simulink model "robot_action"  (R2014b)
settings: Solver=ode45  StartTime=0.0  StopTime=10  FixedStep=1e-4  RelTol=1e-3
values from neighbouring files (symbols this model uses):
  robot_floor_friction_coeff = 0.6    [robot_init.m]
  robot_floor_position_gain = -1e5    (= -100000)    [robot_init.m]
  robot_floor_speed_gain = -1e3    (= -1000)    [robot_init.m]
  robot_gravity = [0 0 -9.80665]    [robot_init.m]
undefined symbols (not defined in the file or in its folder): CM730_acc_center, CM730_acc_gain, CM730_gyro_center, CM730_gyro_gain, CM730_sample_time, FSR_max, FSR_no_load, FSR_sample_time, FSR_scale, MX28_inertia, MX28_Te, X, Y, Z
libraries: sm_lib x158, fl_lib x128, nesl_utility x77
(part 5 of 6)

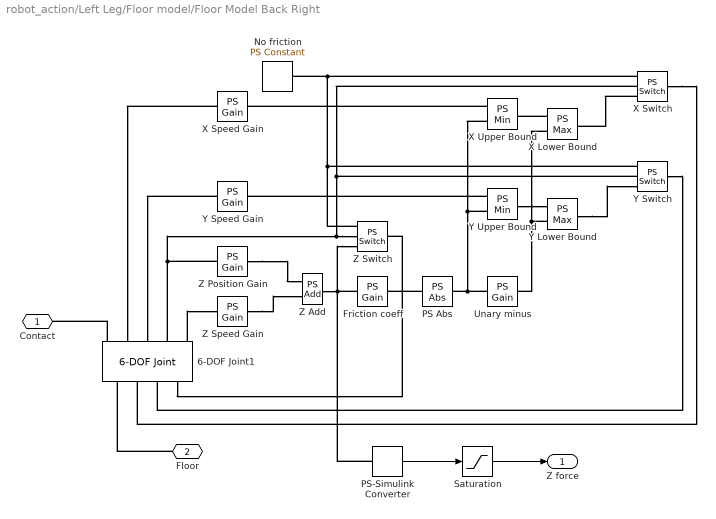
== system robot_action/Left Leg/Floor model/Floor Model Back Right ==
  6-DOF Joint1 : sm_lib/Joints/6-DOF Joint  SenseConstraintForce=off  SenseConstraintForceX=off  SenseConstraintForceY=off  SenseConstraintForceZ=off  SenseConstraintTorque=off  SenseConstraintTorqueX=off  SenseConstraintTorqueY=off  SenseConstraintTorqueZ=off  SenseTotalForce=off  SenseTotalForceX=off  SenseTotalForceY=off  SenseTotalForceZ=off  SenseTotalTorque=off  SenseTotalTorqueX=off  SenseTotalTorqueY=off  SenseTotalTorqueZ=off  CompositeWrenchDir=FollowerOnBase  CompositeWrenchFrame=BaseFrame  PxEquilibriumPosition=0  PxEquilibriumPositionUnits=m  PxSpringStiffness=0  PxSpringStiffnessUnits=N/m  PxDampingCoefficient=0  PxDampingCoefficientUnits=N/(m/s)  PxTorqueActuationMode=InputTorque  PxMotionActuationMode=ComputedMotion  PxSensePosition=off  PxSenseVelocity=on  PxSenseAcceleration=off  PxSenseTorqueForce=off  PxPositionTargetValue=0  PxPositionTargetValueUnits=m  PxPositionTargetSpecify=off  PxPositionTargetPriority=High  PxVelocityTargetValue=0  PxVelocityTargetValueUnits=m/s  PxVelocityTargetSpecify=off  PxVelocityTargetPriority=High  PyEquilibriumPosition=0  PyEquilibriumPositionUnits=m  PySpringStiffness=0  PySpringStiffnessUnits=N/m  PyDampingCoefficient=0  PyDampingCoefficientUnits=N/(m/s)  PyTorqueActuationMode=InputTorque  PyMotionActuationMode=ComputedMotion  PySensePosition=off  PySenseVelocity=on  PySenseAcceleration=off  PySenseTorqueForce=off  PyPositionTargetValue=0  PyPositionTargetValueUnits=m  PyPositionTargetSpecify=off  PyPositionTargetPriority=High  PyVelocityTargetValue=0  PyVelocityTargetValueUnits=m/s  PyVelocityTargetSpecify=off  PyVelocityTargetPriority=High  PzEquilibriumPosition=0  PzEquilibriumPositionUnits=m  PzSpringStiffness=0  PzSpringStiffnessUnits=N/m  PzDampingCoefficient=0  PzDampingCoefficientUnits=N/(m/s)  PzTorqueActuationMode=InputTorque  PzMotionActuationMode=ComputedMotion  PzSensePosition=on  PzSenseVelocity=on  PzSenseAcceleration=off  PzSenseTorqueForce=off  PzPositionTargetValue=0  PzPositionTargetValueUnits=m  PzPositionTargetSpecify=off  PzPositionTargetPriority=High  PzVelocityTargetValue=0  PzVelocityTargetValueUnits=m/s  PzVelocityTargetSpecify=off  PzVelocityTargetPriority=High  SphDefPosRotationMethod=None  SphDefPosRotationAngleUnits=deg  SphDefPosRotationStandardAxis=+Z  SphDefPosRotationAngle=0.0  SphDefPosRotationArbitraryAxis=[0 0 1]  SphDefPosFollAlignAxisA=+X  SphDefPosBaseAlignAxisA=+Y  SphDefPosFollAlignAxisB=+Y  SphDefPosBaseAlignAxisB=+Z  SphDefPosRotationMatrix=[1 0 0; 0 1 0; 0 0 1]  SphEqPosRotationMethod=None  SphEqPosRotationAngleUnits=deg  SphEqPosRotationStandardAxis=+Z  SphEqPosRotationAngle=0.0  SphEqPosRotationArbitraryAxis=[0 0 1]  SphEqPosFollAlignAxisA=+X  SphEqPosBaseAlignAxisA=+Y  SphEqPosFollAlignAxisB=+Y  SphEqPosBaseAlignAxisB=+Z  SphEqPosRotationMatrix=[1 0 0; 0 1 0; 0 0 1]  SphSpringStiffness=0  SphSpringStiffnessUnits=N*m/deg  SphDampingCoefficient=0  SphDampingCoefficientUnits=N*m/(deg/s)  SphActuateTorqueX=off  SphActuateTorqueY=off  SphActuateTorqueZ=off  SphActuateTorque=off  SphTorqueActuationMode=NoTorque  SphMotionActuationMode=ComputedMotion  SphActuationFrame=BaseFrame  SphSensePosition=off  SphSenseVelocityX=off  SphSenseVelocityY=off  SphSenseVelocityZ=off  SphSenseVelocity=off  SphSenseAccelerationX=off  SphSenseAccelerationY=off  SphSenseAccelerationZ=off  SphSenseAcceleration=off  SphSenseTorqueX=off  SphSenseTorqueY=off  SphSenseTorqueZ=off  SphSenseTorqueForce=off  SphSensingFrame=BaseFrame  SphPositionTargetRotationMethod=None  SphPositionTargetRotationAngleUnits=deg  SphPositionTargetRotationStandardAxis=+Z  SphPositionTargetRotationAngle=0.0  SphPositionTargetRotationArbitraryAxis=[0 0 1]  SphPositionTargetFollAlignAxisA=+X  SphPositionTargetBaseAlignAxisA=+Y  SphPositionTargetFollAlignAxisB=+Y  SphPositionTargetBaseAlignAxisB=+Z  SphPositionTargetRotationMatrix=[1 0 0; 0 1 0; 0 0 1]  SphPositionTargetSpecify=off  SphPositionTargetPriority=High  SphVelocityTargetValue=[0 0 0]  SphVelocityTargetValueUnits=deg/s  SphVelocityTargetSpecify=off  SphVelocityTargetPriority=High  SphVelocityTargetInFollowerFrame=on  BlockFunction=simmechanics.library.joints.sixdof_joint
  Friction coeff : fl_lib/Physical Signals/Functions/PS Gain  gain=robot_floor_friction_coeff
  No friction : fl_lib/Physical Signals/Sources/PS Constant  constant=0
  PS Abs : fl_lib/Physical Signals/Nonlinear Operators/PS Abs
  PS-Simulink Converter : nesl_utility/PS-Simulink Converter  PhysicalDomain=network_engine_domain  SubClassName=ps_output  LeftPortType=input  RightPortType=output  PseudoPeriodic=off  Frequencies=[]  Unit=N  AffineConversion=off
  Saturation : Saturate  UpperLimit=+inf  LowerLimit=0
  Unary minus : fl_lib/Physical Signals/Functions/PS Gain  gain=-1
  X Lower Bound : fl_lib/Physical Signals/Nonlinear Operators/PS Max
  X Speed Gain : fl_lib/Physical Signals/Functions/PS Gain  gain=robot_floor_speed_gain
  X Switch : fl_lib/Physical Signals/Nonlinear Operators/PS Switch  Threshold=0
  X Upper Bound : fl_lib/Physical Signals/Nonlinear Operators/PS Min
  Y Lower Bound : fl_lib/Physical Signals/Nonlinear Operators/PS Max
  Y Speed Gain : fl_lib/Physical Signals/Functions/PS Gain  gain=robot_floor_speed_gain
  Y Switch : fl_lib/Physical Signals/Nonlinear Operators/PS Switch  Threshold=0
  Y Upper Bound : fl_lib/Physical Signals/Nonlinear Operators/PS Min
  Z Add : fl_lib/Physical Signals/Functions/PS Add
  Z Position Gain : fl_lib/Physical Signals/Functions/PS Gain  gain=robot_floor_position_gain
  Z Speed Gain : fl_lib/Physical Signals/Functions/PS Gain  gain=robot_floor_speed_gain
  Z Switch : fl_lib/Physical Signals/Nonlinear Operators/PS Switch  Threshold=0
  Contact : PMIOPort  Port=1  Side=Left
  Floor : PMIOPort  Port=2  Side=Right
  Z force : Outport
  wires:
  PS-Simulink Converter/1 -> Saturation/1
  Saturation/1 -> Z force/1
  connections:
  Floor/RConn1 -- 6-DOF Joint1/LConn1
  6-DOF Joint1/RConn1 -- Contact/RConn1
  No friction/RConn1 -- Y Switch/LConn1 -- Z Switch/LConn1 -- X Switch/LConn1
  Z Position Gain/RConn1 -- Z Add/LConn1
  Z Switch/LConn3 -- Z Add/RConn1 -- Friction coeff/LConn1 -- PS-Simulink Converter/LConn1
  Z Speed Gain/RConn1 -- Z Add/LConn2
  6-DOF Joint1/RConn5 -- Z Speed Gain/LConn1
  6-DOF Joint1/LConn4 -- Z Switch/RConn1
  Z Switch/LConn2 -- Z Position Gain/LConn1 -- 6-DOF Joint1/RConn4 -- X Switch/LConn2 -- Y Switch/LConn2
  Y Switch/RConn1 -- 6-DOF Joint1/LConn3
  Y Speed Gain/LConn1 -- 6-DOF Joint1/RConn3
  PS Abs/LConn1 -- Friction coeff/RConn1
  PS Abs/RConn1 -- Unary minus/LConn1 -- X Upper Bound/LConn2 -- Y Upper Bound/LConn2
  Y Upper Bound/RConn1 -- Y Lower Bound/LConn1
  Y Lower Bound/LConn2 -- Unary minus/RConn1 -- X Lower Bound/LConn2
  Y Lower Bound/RConn1 -- Y Switch/LConn3
  Y Upper Bound/LConn1 -- Y Speed Gain/RConn1
  X Speed Gain/LConn1 -- 6-DOF Joint1/RConn2
  X Upper Bound/LConn1 -- X Speed Gain/RConn1
  X Lower Bound/LConn1 -- X Upper Bound/RConn1
  X Switch/LConn3 -- X Lower Bound/RConn1
  X Switch/RConn1 -- 6-DOF Joint1/LConn2

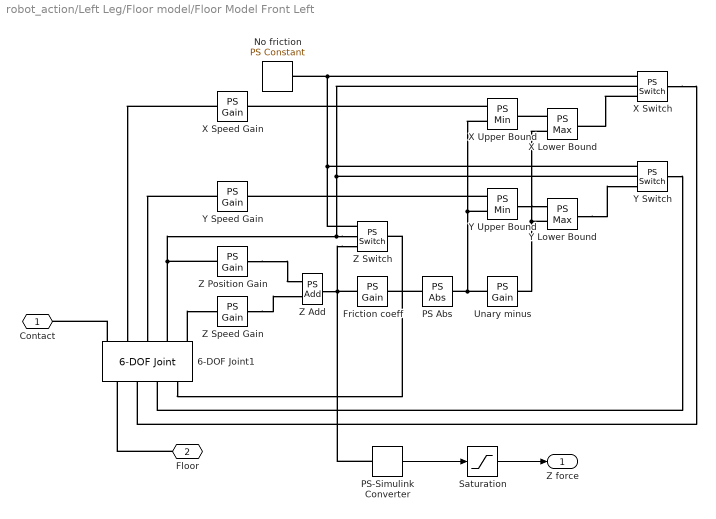
== system robot_action/Left Leg/Floor model/Floor Model Front Left ==
  6-DOF Joint1 : sm_lib/Joints/6-DOF Joint  SenseConstraintForce=off  SenseConstraintForceX=off  SenseConstraintForceY=off  SenseConstraintForceZ=off  SenseConstraintTorque=off  SenseConstraintTorqueX=off  SenseConstraintTorqueY=off  SenseConstraintTorqueZ=off  SenseTotalForce=off  SenseTotalForceX=off  SenseTotalForceY=off  SenseTotalForceZ=off  SenseTotalTorque=off  SenseTotalTorqueX=off  SenseTotalTorqueY=off  SenseTotalTorqueZ=off  CompositeWrenchDir=FollowerOnBase  CompositeWrenchFrame=BaseFrame  PxEquilibriumPosition=0  PxEquilibriumPositionUnits=m  PxSpringStiffness=0  PxSpringStiffnessUnits=N/m  PxDampingCoefficient=0  PxDampingCoefficientUnits=N/(m/s)  PxTorqueActuationMode=InputTorque  PxMotionActuationMode=ComputedMotion  PxSensePosition=off  PxSenseVelocity=on  PxSenseAcceleration=off  PxSenseTorqueForce=off  PxPositionTargetValue=0  PxPositionTargetValueUnits=m  PxPositionTargetSpecify=off  PxPositionTargetPriority=High  PxVelocityTargetValue=0  PxVelocityTargetValueUnits=m/s  PxVelocityTargetSpecify=off  PxVelocityTargetPriority=High  PyEquilibriumPosition=0  PyEquilibriumPositionUnits=m  PySpringStiffness=0  PySpringStiffnessUnits=N/m  PyDampingCoefficient=0  PyDampingCoefficientUnits=N/(m/s)  PyTorqueActuationMode=InputTorque  PyMotionActuationMode=ComputedMotion  PySensePosition=off  PySenseVelocity=on  PySenseAcceleration=off  PySenseTorqueForce=off  PyPositionTargetValue=0  PyPositionTargetValueUnits=m  PyPositionTargetSpecify=off  PyPositionTargetPriority=High  PyVelocityTargetValue=0  PyVelocityTargetValueUnits=m/s  PyVelocityTargetSpecify=off  PyVelocityTargetPriority=High  PzEquilibriumPosition=0  PzEquilibriumPositionUnits=m  PzSpringStiffness=0  PzSpringStiffnessUnits=N/m  PzDampingCoefficient=0  PzDampingCoefficientUnits=N/(m/s)  PzTorqueActuationMode=InputTorque  PzMotionActuationMode=ComputedMotion  PzSensePosition=on  PzSenseVelocity=on  PzSenseAcceleration=off  PzSenseTorqueForce=off  PzPositionTargetValue=0  PzPositionTargetValueUnits=m  PzPositionTargetSpecify=off  PzPositionTargetPriority=High  PzVelocityTargetValue=0  PzVelocityTargetValueUnits=m/s  PzVelocityTargetSpecify=off  PzVelocityTargetPriority=High  SphDefPosRotationMethod=None  SphDefPosRotationAngleUnits=deg  SphDefPosRotationStandardAxis=+Z  SphDefPosRotationAngle=0.0  SphDefPosRotationArbitraryAxis=[0 0 1]  SphDefPosFollAlignAxisA=+X  SphDefPosBaseAlignAxisA=+Y  SphDefPosFollAlignAxisB=+Y  SphDefPosBaseAlignAxisB=+Z  SphDefPosRotationMatrix=[1 0 0; 0 1 0; 0 0 1]  SphEqPosRotationMethod=None  SphEqPosRotationAngleUnits=deg  SphEqPosRotationStandardAxis=+Z  SphEqPosRotationAngle=0.0  SphEqPosRotationArbitraryAxis=[0 0 1]  SphEqPosFollAlignAxisA=+X  SphEqPosBaseAlignAxisA=+Y  SphEqPosFollAlignAxisB=+Y  SphEqPosBaseAlignAxisB=+Z  SphEqPosRotationMatrix=[1 0 0; 0 1 0; 0 0 1]  SphSpringStiffness=0  SphSpringStiffnessUnits=N*m/deg  SphDampingCoefficient=0  SphDampingCoefficientUnits=N*m/(deg/s)  SphActuateTorqueX=off  SphActuateTorqueY=off  SphActuateTorqueZ=off  SphActuateTorque=off  SphTorqueActuationMode=NoTorque  SphMotionActuationMode=ComputedMotion  SphActuationFrame=BaseFrame  SphSensePosition=off  SphSenseVelocityX=off  SphSenseVelocityY=off  SphSenseVelocityZ=off  SphSenseVelocity=off  SphSenseAccelerationX=off  SphSenseAccelerationY=off  SphSenseAccelerationZ=off  SphSenseAcceleration=off  SphSenseTorqueX=off  SphSenseTorqueY=off  SphSenseTorqueZ=off  SphSenseTorqueForce=off  SphSensingFrame=BaseFrame  SphPositionTargetRotationMethod=None  SphPositionTargetRotationAngleUnits=deg  SphPositionTargetRotationStandardAxis=+Z  SphPositionTargetRotationAngle=0.0  SphPositionTargetRotationArbitraryAxis=[0 0 1]  SphPositionTargetFollAlignAxisA=+X  SphPositionTargetBaseAlignAxisA=+Y  SphPositionTargetFollAlignAxisB=+Y  SphPositionTargetBaseAlignAxisB=+Z  SphPositionTargetRotationMatrix=[1 0 0; 0 1 0; 0 0 1]  SphPositionTargetSpecify=off  SphPositionTargetPriority=High  SphVelocityTargetValue=[0 0 0]  SphVelocityTargetValueUnits=deg/s  SphVelocityTargetSpecify=off  SphVelocityTargetPriority=High  SphVelocityTargetInFollowerFrame=on  BlockFunction=simmechanics.library.joints.sixdof_joint
  Friction coeff : fl_lib/Physical Signals/Functions/PS Gain  gain=robot_floor_friction_coeff
  No friction : fl_lib/Physical Signals/Sources/PS Constant  constant=0
  PS Abs : fl_lib/Physical Signals/Nonlinear Operators/PS Abs
  PS-Simulink Converter : nesl_utility/PS-Simulink Converter  PhysicalDomain=network_engine_domain  SubClassName=ps_output  LeftPortType=input  RightPortType=output  PseudoPeriodic=off  Frequencies=[]  Unit=N  AffineConversion=off
  Saturation : Saturate  UpperLimit=+inf  LowerLimit=0
  Unary minus : fl_lib/Physical Signals/Functions/PS Gain  gain=-1
  X Lower Bound : fl_lib/Physical Signals/Nonlinear Operators/PS Max
  X Speed Gain : fl_lib/Physical Signals/Functions/PS Gain  gain=robot_floor_speed_gain
  X Switch : fl_lib/Physical Signals/Nonlinear Operators/PS Switch  Threshold=0
  X Upper Bound : fl_lib/Physical Signals/Nonlinear Operators/PS Min
  Y Lower Bound : fl_lib/Physical Signals/Nonlinear Operators/PS Max
  Y Speed Gain : fl_lib/Physical Signals/Functions/PS Gain  gain=robot_floor_speed_gain
  Y Switch : fl_lib/Physical Signals/Nonlinear Operators/PS Switch  Threshold=0
  Y Upper Bound : fl_lib/Physical Signals/Nonlinear Operators/PS Min
  Z Add : fl_lib/Physical Signals/Functions/PS Add
  Z Position Gain : fl_lib/Physical Signals/Functions/PS Gain  gain=robot_floor_position_gain
  Z Speed Gain : fl_lib/Physical Signals/Functions/PS Gain  gain=robot_floor_speed_gain
  Z Switch : fl_lib/Physical Signals/Nonlinear Operators/PS Switch  Threshold=0
  Contact : PMIOPort  Port=1  Side=Left
  Floor : PMIOPort  Port=2  Side=Right
  Z force : Outport
  wires:
  PS-Simulink Converter/1 -> Saturation/1
  Saturation/1 -> Z force/1
  connections:
  Floor/RConn1 -- 6-DOF Joint1/LConn1
  6-DOF Joint1/RConn1 -- Contact/RConn1
  No friction/RConn1 -- Y Switch/LConn1 -- Z Switch/LConn1 -- X Switch/LConn1
  Z Position Gain/RConn1 -- Z Add/LConn1
  Z Switch/LConn3 -- PS-Simulink Converter/LConn1 -- Z Add/RConn1 -- Friction coeff/LConn1
  Z Speed Gain/RConn1 -- Z Add/LConn2
  6-DOF Joint1/RConn5 -- Z Speed Gain/LConn1
  6-DOF Joint1/LConn4 -- Z Switch/RConn1
  Z Switch/LConn2 -- Z Position Gain/LConn1 -- 6-DOF Joint1/RConn4 -- X Switch/LConn2 -- Y Switch/LConn2
  Y Switch/RConn1 -- 6-DOF Joint1/LConn3
  Y Speed Gain/LConn1 -- 6-DOF Joint1/RConn3
  PS Abs/LConn1 -- Friction coeff/RConn1
  PS Abs/RConn1 -- Unary minus/LConn1 -- X Upper Bound/LConn2 -- Y Upper Bound/LConn2
  Y Upper Bound/RConn1 -- Y Lower Bound/LConn1
  Y Lower Bound/LConn2 -- Unary minus/RConn1 -- X Lower Bound/LConn2
  Y Lower Bound/RConn1 -- Y Switch/LConn3
  Y Upper Bound/LConn1 -- Y Speed Gain/RConn1
  X Speed Gain/LConn1 -- 6-DOF Joint1/RConn2
  X Upper Bound/LConn1 -- X Speed Gain/RConn1
  X Lower Bound/LConn1 -- X Upper Bound/RConn1
  X Switch/LConn3 -- X Lower Bound/RConn1
  X Switch/RConn1 -- 6-DOF Joint1/LConn2

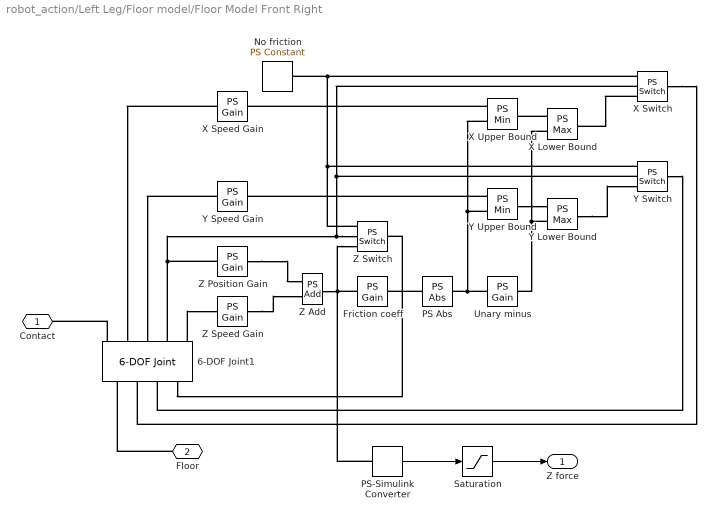
== system robot_action/Left Leg/Floor model/Floor Model Front Right ==
  6-DOF Joint1 : sm_lib/Joints/6-DOF Joint  SenseConstraintForce=off  SenseConstraintForceX=off  SenseConstraintForceY=off  SenseConstraintForceZ=off  SenseConstraintTorque=off  SenseConstraintTorqueX=off  SenseConstraintTorqueY=off  SenseConstraintTorqueZ=off  SenseTotalForce=off  SenseTotalForceX=off  SenseTotalForceY=off  SenseTotalForceZ=off  SenseTotalTorque=off  SenseTotalTorqueX=off  SenseTotalTorqueY=off  SenseTotalTorqueZ=off  CompositeWrenchDir=FollowerOnBase  CompositeWrenchFrame=BaseFrame  PxEquilibriumPosition=0  PxEquilibriumPositionUnits=m  PxSpringStiffness=0  PxSpringStiffnessUnits=N/m  PxDampingCoefficient=0  PxDampingCoefficientUnits=N/(m/s)  PxTorqueActuationMode=InputTorque  PxMotionActuationMode=ComputedMotion  PxSensePosition=off  PxSenseVelocity=on  PxSenseAcceleration=off  PxSenseTorqueForce=off  PxPositionTargetValue=0  PxPositionTargetValueUnits=m  PxPositionTargetSpecify=off  PxPositionTargetPriority=High  PxVelocityTargetValue=0  PxVelocityTargetValueUnits=m/s  PxVelocityTargetSpecify=off  PxVelocityTargetPriority=High  PyEquilibriumPosition=0  PyEquilibriumPositionUnits=m  PySpringStiffness=0  PySpringStiffnessUnits=N/m  PyDampingCoefficient=0  PyDampingCoefficientUnits=N/(m/s)  PyTorqueActuationMode=InputTorque  PyMotionActuationMode=ComputedMotion  PySensePosition=off  PySenseVelocity=on  PySenseAcceleration=off  PySenseTorqueForce=off  PyPositionTargetValue=0  PyPositionTargetValueUnits=m  PyPositionTargetSpecify=off  PyPositionTargetPriority=High  PyVelocityTargetValue=0  PyVelocityTargetValueUnits=m/s  PyVelocityTargetSpecify=off  PyVelocityTargetPriority=High  PzEquilibriumPosition=0  PzEquilibriumPositionUnits=m  PzSpringStiffness=0  PzSpringStiffnessUnits=N/m  PzDampingCoefficient=0  PzDampingCoefficientUnits=N/(m/s)  PzTorqueActuationMode=InputTorque  PzMotionActuationMode=ComputedMotion  PzSensePosition=on  PzSenseVelocity=on  PzSenseAcceleration=off  PzSenseTorqueForce=off  PzPositionTargetValue=0  PzPositionTargetValueUnits=m  PzPositionTargetSpecify=off  PzPositionTargetPriority=High  PzVelocityTargetValue=0  PzVelocityTargetValueUnits=m/s  PzVelocityTargetSpecify=off  PzVelocityTargetPriority=High  SphDefPosRotationMethod=None  SphDefPosRotationAngleUnits=deg  SphDefPosRotationStandardAxis=+Z  SphDefPosRotationAngle=0.0  SphDefPosRotationArbitraryAxis=[0 0 1]  SphDefPosFollAlignAxisA=+X  SphDefPosBaseAlignAxisA=+Y  SphDefPosFollAlignAxisB=+Y  SphDefPosBaseAlignAxisB=+Z  SphDefPosRotationMatrix=[1 0 0; 0 1 0; 0 0 1]  SphEqPosRotationMethod=None  SphEqPosRotationAngleUnits=deg  SphEqPosRotationStandardAxis=+Z  SphEqPosRotationAngle=0.0  SphEqPosRotationArbitraryAxis=[0 0 1]  SphEqPosFollAlignAxisA=+X  SphEqPosBaseAlignAxisA=+Y  SphEqPosFollAlignAxisB=+Y  SphEqPosBaseAlignAxisB=+Z  SphEqPosRotationMatrix=[1 0 0; 0 1 0; 0 0 1]  SphSpringStiffness=0  SphSpringStiffnessUnits=N*m/deg  SphDampingCoefficient=0  SphDampingCoefficientUnits=N*m/(deg/s)  SphActuateTorqueX=off  SphActuateTorqueY=off  SphActuateTorqueZ=off  SphActuateTorque=off  SphTorqueActuationMode=NoTorque  SphMotionActuationMode=ComputedMotion  SphActuationFrame=BaseFrame  SphSensePosition=off  SphSenseVelocityX=off  SphSenseVelocityY=off  SphSenseVelocityZ=off  SphSenseVelocity=off  SphSenseAccelerationX=off  SphSenseAccelerationY=off  SphSenseAccelerationZ=off  SphSenseAcceleration=off  SphSenseTorqueX=off  SphSenseTorqueY=off  SphSenseTorqueZ=off  SphSenseTorqueForce=off  SphSensingFrame=BaseFrame  SphPositionTargetRotationMethod=None  SphPositionTargetRotationAngleUnits=deg  SphPositionTargetRotationStandardAxis=+Z  SphPositionTargetRotationAngle=0.0  SphPositionTargetRotationArbitraryAxis=[0 0 1]  SphPositionTargetFollAlignAxisA=+X  SphPositionTargetBaseAlignAxisA=+Y  SphPositionTargetFollAlignAxisB=+Y  SphPositionTargetBaseAlignAxisB=+Z  SphPositionTargetRotationMatrix=[1 0 0; 0 1 0; 0 0 1]  SphPositionTargetSpecify=off  SphPositionTargetPriority=High  SphVelocityTargetValue=[0 0 0]  SphVelocityTargetValueUnits=deg/s  SphVelocityTargetSpecify=off  SphVelocityTargetPriority=High  SphVelocityTargetInFollowerFrame=on  BlockFunction=simmechanics.library.joints.sixdof_joint
  Friction coeff : fl_lib/Physical Signals/Functions/PS Gain  gain=robot_floor_friction_coeff
  No friction : fl_lib/Physical Signals/Sources/PS Constant  constant=0
  PS Abs : fl_lib/Physical Signals/Nonlinear Operators/PS Abs
  PS-Simulink Converter : nesl_utility/PS-Simulink Converter  PhysicalDomain=network_engine_domain  SubClassName=ps_output  LeftPortType=input  RightPortType=output  PseudoPeriodic=off  Frequencies=[]  Unit=N  AffineConversion=off
  Saturation : Saturate  UpperLimit=+inf  LowerLimit=0
  Unary minus : fl_lib/Physical Signals/Functions/PS Gain  gain=-1
  X Lower Bound : fl_lib/Physical Signals/Nonlinear Operators/PS Max
  X Speed Gain : fl_lib/Physical Signals/Functions/PS Gain  gain=robot_floor_speed_gain
  X Switch : fl_lib/Physical Signals/Nonlinear Operators/PS Switch  Threshold=0
  X Upper Bound : fl_lib/Physical Signals/Nonlinear Operators/PS Min
  Y Lower Bound : fl_lib/Physical Signals/Nonlinear Operators/PS Max
  Y Speed Gain : fl_lib/Physical Signals/Functions/PS Gain  gain=robot_floor_speed_gain
  Y Switch : fl_lib/Physical Signals/Nonlinear Operators/PS Switch  Threshold=0
  Y Upper Bound : fl_lib/Physical Signals/Nonlinear Operators/PS Min
  Z Add : fl_lib/Physical Signals/Functions/PS Add
  Z Position Gain : fl_lib/Physical Signals/Functions/PS Gain  gain=robot_floor_position_gain
  Z Speed Gain : fl_lib/Physical Signals/Functions/PS Gain  gain=robot_floor_speed_gain
  Z Switch : fl_lib/Physical Signals/Nonlinear Operators/PS Switch  Threshold=0
  Contact : PMIOPort  Port=1  Side=Left
  Floor : PMIOPort  Port=2  Side=Right
  Z force : Outport
  wires:
  PS-Simulink Converter/1 -> Saturation/1
  Saturation/1 -> Z force/1
  connections:
  Floor/RConn1 -- 6-DOF Joint1/LConn1
  6-DOF Joint1/RConn1 -- Contact/RConn1
  No friction/RConn1 -- Y Switch/LConn1 -- Z Switch/LConn1 -- X Switch/LConn1
  Z Position Gain/RConn1 -- Z Add/LConn1
  Z Switch/LConn3 -- Z Add/RConn1 -- Friction coeff/LConn1 -- PS-Simulink Converter/LConn1
  Z Speed Gain/RConn1 -- Z Add/LConn2
  6-DOF Joint1/RConn5 -- Z Speed Gain/LConn1
  6-DOF Joint1/LConn4 -- Z Switch/RConn1
  Z Switch/LConn2 -- Z Position Gain/LConn1 -- 6-DOF Joint1/RConn4 -- X Switch/LConn2 -- Y Switch/LConn2
  Y Switch/RConn1 -- 6-DOF Joint1/LConn3
  Y Speed Gain/LConn1 -- 6-DOF Joint1/RConn3
  PS Abs/LConn1 -- Friction coeff/RConn1
  PS Abs/RConn1 -- Unary minus/LConn1 -- X Upper Bound/LConn2 -- Y Upper Bound/LConn2
  Y Upper Bound/RConn1 -- Y Lower Bound/LConn1
  Y Lower Bound/LConn2 -- Unary minus/RConn1 -- X Lower Bound/LConn2
  Y Lower Bound/RConn1 -- Y Switch/LConn3
  Y Upper Bound/LConn1 -- Y Speed Gain/RConn1
  X Speed Gain/LConn1 -- 6-DOF Joint1/RConn2
  X Upper Bound/LConn1 -- X Speed Gain/RConn1
  X Lower Bound/LConn1 -- X Upper Bound/RConn1
  X Switch/LConn3 -- X Lower Bound/RConn1
  X Switch/RConn1 -- 6-DOF Joint1/LConn2

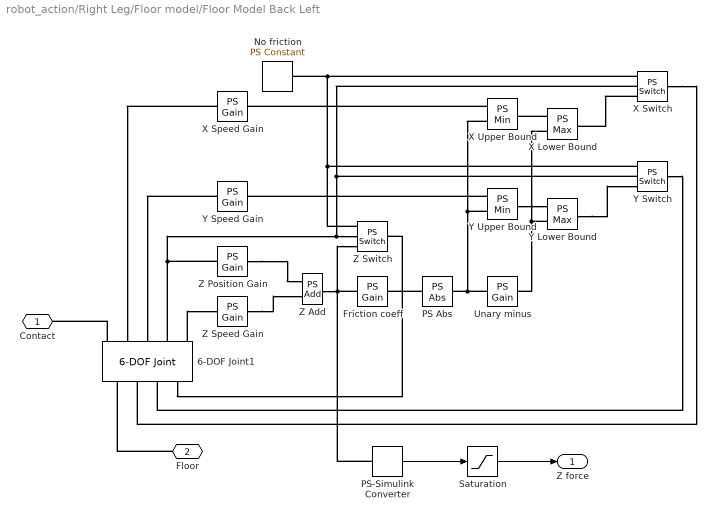
== system robot_action/Right Leg/Floor model/Floor Model Back Left ==
  6-DOF Joint1 : sm_lib/Joints/6-DOF Joint  SenseConstraintForce=off  SenseConstraintForceX=off  SenseConstraintForceY=off  SenseConstraintForceZ=off  SenseConstraintTorque=off  SenseConstraintTorqueX=off  SenseConstraintTorqueY=off  SenseConstraintTorqueZ=off  SenseTotalForce=off  SenseTotalForceX=off  SenseTotalForceY=off  SenseTotalForceZ=off  SenseTotalTorque=off  SenseTotalTorqueX=off  SenseTotalTorqueY=off  SenseTotalTorqueZ=off  CompositeWrenchDir=FollowerOnBase  CompositeWrenchFrame=BaseFrame  PxEquilibriumPosition=0  PxEquilibriumPositionUnits=m  PxSpringStiffness=0  PxSpringStiffnessUnits=N/m  PxDampingCoefficient=0  PxDampingCoefficientUnits=N/(m/s)  PxTorqueActuationMode=InputTorque  PxMotionActuationMode=ComputedMotion  PxSensePosition=off  PxSenseVelocity=on  PxSenseAcceleration=off  PxSenseTorqueForce=off  PxPositionTargetValue=0  PxPositionTargetValueUnits=m  PxPositionTargetSpecify=off  PxPositionTargetPriority=High  PxVelocityTargetValue=0  PxVelocityTargetValueUnits=m/s  PxVelocityTargetSpecify=off  PxVelocityTargetPriority=High  PyEquilibriumPosition=0  PyEquilibriumPositionUnits=m  PySpringStiffness=0  PySpringStiffnessUnits=N/m  PyDampingCoefficient=0  PyDampingCoefficientUnits=N/(m/s)  PyTorqueActuationMode=InputTorque  PyMotionActuationMode=ComputedMotion  PySensePosition=off  PySenseVelocity=on  PySenseAcceleration=off  PySenseTorqueForce=off  PyPositionTargetValue=0  PyPositionTargetValueUnits=m  PyPositionTargetSpecify=off  PyPositionTargetPriority=High  PyVelocityTargetValue=0  PyVelocityTargetValueUnits=m/s  PyVelocityTargetSpecify=off  PyVelocityTargetPriority=High  PzEquilibriumPosition=0  PzEquilibriumPositionUnits=m  PzSpringStiffness=0  PzSpringStiffnessUnits=N/m  PzDampingCoefficient=0  PzDampingCoefficientUnits=N/(m/s)  PzTorqueActuationMode=InputTorque  PzMotionActuationMode=ComputedMotion  PzSensePosition=on  PzSenseVelocity=on  PzSenseAcceleration=off  PzSenseTorqueForce=off  PzPositionTargetValue=0  PzPositionTargetValueUnits=m  PzPositionTargetSpecify=off  PzPositionTargetPriority=High  PzVelocityTargetValue=0  PzVelocityTargetValueUnits=m/s  PzVelocityTargetSpecify=off  PzVelocityTargetPriority=High  SphDefPosRotationMethod=None  SphDefPosRotationAngleUnits=deg  SphDefPosRotationStandardAxis=+Z  SphDefPosRotationAngle=0.0  SphDefPosRotationArbitraryAxis=[0 0 1]  SphDefPosFollAlignAxisA=+X  SphDefPosBaseAlignAxisA=+Y  SphDefPosFollAlignAxisB=+Y  SphDefPosBaseAlignAxisB=+Z  SphDefPosRotationMatrix=[1 0 0; 0 1 0; 0 0 1]  SphEqPosRotationMethod=None  SphEqPosRotationAngleUnits=deg  SphEqPosRotationStandardAxis=+Z  SphEqPosRotationAngle=0.0  SphEqPosRotationArbitraryAxis=[0 0 1]  SphEqPosFollAlignAxisA=+X  SphEqPosBaseAlignAxisA=+Y  SphEqPosFollAlignAxisB=+Y  SphEqPosBaseAlignAxisB=+Z  SphEqPosRotationMatrix=[1 0 0; 0 1 0; 0 0 1]  SphSpringStiffness=0  SphSpringStiffnessUnits=N*m/deg  SphDampingCoefficient=0  SphDampingCoefficientUnits=N*m/(deg/s)  SphActuateTorqueX=off  SphActuateTorqueY=off  SphActuateTorqueZ=off  SphActuateTorque=off  SphTorqueActuationMode=NoTorque  SphMotionActuationMode=ComputedMotion  SphActuationFrame=BaseFrame  SphSensePosition=off  SphSenseVelocityX=off  SphSenseVelocityY=off  SphSenseVelocityZ=off  SphSenseVelocity=off  SphSenseAccelerationX=off  SphSenseAccelerationY=off  SphSenseAccelerationZ=off  SphSenseAcceleration=off  SphSenseTorqueX=off  SphSenseTorqueY=off  SphSenseTorqueZ=off  SphSenseTorqueForce=off  SphSensingFrame=BaseFrame  SphPositionTargetRotationMethod=None  SphPositionTargetRotationAngleUnits=deg  SphPositionTargetRotationStandardAxis=+Z  SphPositionTargetRotationAngle=0.0  SphPositionTargetRotationArbitraryAxis=[0 0 1]  SphPositionTargetFollAlignAxisA=+X  SphPositionTargetBaseAlignAxisA=+Y  SphPositionTargetFollAlignAxisB=+Y  SphPositionTargetBaseAlignAxisB=+Z  SphPositionTargetRotationMatrix=[1 0 0; 0 1 0; 0 0 1]  SphPositionTargetSpecify=off  SphPositionTargetPriority=High  SphVelocityTargetValue=[0 0 0]  SphVelocityTargetValueUnits=deg/s  SphVelocityTargetSpecify=off  SphVelocityTargetPriority=High  SphVelocityTargetInFollowerFrame=on  BlockFunction=simmechanics.library.joints.sixdof_joint
  Friction coeff : fl_lib/Physical Signals/Functions/PS Gain  gain=robot_floor_friction_coeff
  No friction : fl_lib/Physical Signals/Sources/PS Constant  constant=0
  PS Abs : fl_lib/Physical Signals/Nonlinear Operators/PS Abs
  PS-Simulink Converter : nesl_utility/PS-Simulink Converter  PhysicalDomain=network_engine_domain  SubClassName=ps_output  LeftPortType=input  RightPortType=output  PseudoPeriodic=off  Frequencies=[]  Unit=N  AffineConversion=off
  Saturation : Saturate  UpperLimit=+inf  LowerLimit=0
  Unary minus : fl_lib/Physical Signals/Functions/PS Gain  gain=-1
  X Lower Bound : fl_lib/Physical Signals/Nonlinear Operators/PS Max
  X Speed Gain : fl_lib/Physical Signals/Functions/PS Gain  gain=robot_floor_speed_gain
  X Switch : fl_lib/Physical Signals/Nonlinear Operators/PS Switch  Threshold=0
  X Upper Bound : fl_lib/Physical Signals/Nonlinear Operators/PS Min
  Y Lower Bound : fl_lib/Physical Signals/Nonlinear Operators/PS Max
  Y Speed Gain : fl_lib/Physical Signals/Functions/PS Gain  gain=robot_floor_speed_gain
  Y Switch : fl_lib/Physical Signals/Nonlinear Operators/PS Switch  Threshold=0
  Y Upper Bound : fl_lib/Physical Signals/Nonlinear Operators/PS Min
  Z Add : fl_lib/Physical Signals/Functions/PS Add
  Z Position Gain : fl_lib/Physical Signals/Functions/PS Gain  gain=robot_floor_position_gain
  Z Speed Gain : fl_lib/Physical Signals/Functions/PS Gain  gain=robot_floor_speed_gain
  Z Switch : fl_lib/Physical Signals/Nonlinear Operators/PS Switch  Threshold=0
  Contact : PMIOPort  Port=1  Side=Left
  Floor : PMIOPort  Port=2  Side=Right
  Z force : Outport
  wires:
  PS-Simulink Converter/1 -> Saturation/1
  Saturation/1 -> Z force/1
  connections:
  Floor/RConn1 -- 6-DOF Joint1/LConn1
  6-DOF Joint1/RConn1 -- Contact/RConn1
  No friction/RConn1 -- Y Switch/LConn1 -- Z Switch/LConn1 -- X Switch/LConn1
  Z Position Gain/RConn1 -- Z Add/LConn1
  Z Switch/LConn3 -- Z Add/RConn1 -- Friction coeff/LConn1 -- PS-Simulink Converter/LConn1
  Z Speed Gain/RConn1 -- Z Add/LConn2
  6-DOF Joint1/RConn5 -- Z Speed Gain/LConn1
  6-DOF Joint1/LConn4 -- Z Switch/RConn1
  Z Switch/LConn2 -- Z Position Gain/LConn1 -- 6-DOF Joint1/RConn4 -- X Switch/LConn2 -- Y Switch/LConn2
  Y Switch/RConn1 -- 6-DOF Joint1/LConn3
  Y Speed Gain/LConn1 -- 6-DOF Joint1/RConn3
  PS Abs/LConn1 -- Friction coeff/RConn1
  PS Abs/RConn1 -- Unary minus/LConn1 -- X Upper Bound/LConn2 -- Y Upper Bound/LConn2
  Y Upper Bound/RConn1 -- Y Lower Bound/LConn1
  Y Lower Bound/LConn2 -- Unary minus/RConn1 -- X Lower Bound/LConn2
  Y Lower Bound/RConn1 -- Y Switch/LConn3
  Y Upper Bound/LConn1 -- Y Speed Gain/RConn1
  X Speed Gain/LConn1 -- 6-DOF Joint1/RConn2
  X Upper Bound/LConn1 -- X Speed Gain/RConn1
  X Lower Bound/LConn1 -- X Upper Bound/RConn1
  X Switch/LConn3 -- X Lower Bound/RConn1
  X Switch/RConn1 -- 6-DOF Joint1/LConn2

== system robot_action/Right Leg/Floor model/Floor Model Back Right ==
  6-DOF Joint1 : sm_lib/Joints/6-DOF Joint  SenseConstraintForce=off  SenseConstraintForceX=off  SenseConstraintForceY=off  SenseConstraintForceZ=off  SenseConstraintTorque=off  SenseConstraintTorqueX=off  SenseConstraintTorqueY=off  SenseConstraintTorqueZ=off  SenseTotalForce=off  SenseTotalForceX=off  SenseTotalForceY=off  SenseTotalForceZ=off  SenseTotalTorque=off  SenseTotalTorqueX=off  SenseTotalTorqueY=off  SenseTotalTorqueZ=off  CompositeWrenchDir=FollowerOnBase  CompositeWrenchFrame=BaseFrame  PxEquilibriumPosition=0  PxEquilibriumPositionUnits=m  PxSpringStiffness=0  PxSpringStiffnessUnits=N/m  PxDampingCoefficient=0  PxDampingCoefficientUnits=N/(m/s)  PxTorqueActuationMode=InputTorque  PxMotionActuationMode=ComputedMotion  PxSensePosition=off  PxSenseVelocity=on  PxSenseAcceleration=off  PxSenseTorqueForce=off  PxPositionTargetValue=0  PxPositionTargetValueUnits=m  PxPositionTargetSpecify=off  PxPositionTargetPriority=High  PxVelocityTargetValue=0  PxVelocityTargetValueUnits=m/s  PxVelocityTargetSpecify=off  PxVelocityTargetPriority=High  PyEquilibriumPosition=0  PyEquilibriumPositionUnits=m  PySpringStiffness=0  PySpringStiffnessUnits=N/m  PyDampingCoefficient=0  PyDampingCoefficientUnits=N/(m/s)  PyTorqueActuationMode=InputTorque  PyMotionActuationMode=ComputedMotion  PySensePosition=off  PySenseVelocity=on  PySenseAcceleration=off  PySenseTorqueForce=off  PyPositionTargetValue=0  PyPositionTargetValueUnits=m  PyPositionTargetSpecify=off  PyPositionTargetPriority=High  PyVelocityTargetValue=0  PyVelocityTargetValueUnits=m/s  PyVelocityTargetSpecify=off  PyVelocityTargetPriority=High  PzEquilibriumPosition=0  PzEquilibriumPositionUnits=m  PzSpringStiffness=0  PzSpringStiffnessUnits=N/m  PzDampingCoefficient=0  PzDampingCoefficientUnits=N/(m/s)  PzTorqueActuationMode=InputTorque  PzMotionActuationMode=ComputedMotion  PzSensePosition=on  PzSenseVelocity=on  PzSenseAcceleration=off  PzSenseTorqueForce=off  PzPositionTargetValue=0  PzPositionTargetValueUnits=m  PzPositionTargetSpecify=off  PzPositionTargetPriority=High  PzVelocityTargetValue=0  PzVelocityTargetValueUnits=m/s  PzVelocityTargetSpecify=off  PzVelocityTargetPriority=High  SphDefPosRotationMethod=None  SphDefPosRotationAngleUnits=deg  SphDefPosRotationStandardAxis=+Z  SphDefPosRotationAngle=0.0  SphDefPosRotationArbitraryAxis=[0 0 1]  SphDefPosFollAlignAxisA=+X  SphDefPosBaseAlignAxisA=+Y  SphDefPosFollAlignAxisB=+Y  SphDefPosBaseAlignAxisB=+Z  SphDefPosRotationMatrix=[1 0 0; 0 1 0; 0 0 1]  SphEqPosRotationMethod=None  SphEqPosRotationAngleUnits=deg  SphEqPosRotationStandardAxis=+Z  SphEqPosRotationAngle=0.0  SphEqPosRotationArbitraryAxis=[0 0 1]  SphEqPosFollAlignAxisA=+X  SphEqPosBaseAlignAxisA=+Y  SphEqPosFollAlignAxisB=+Y  SphEqPosBaseAlignAxisB=+Z  SphEqPosRotationMatrix=[1 0 0; 0 1 0; 0 0 1]  SphSpringStiffness=0  SphSpringStiffnessUnits=N*m/deg  SphDampingCoefficient=0  SphDampingCoefficientUnits=N*m/(deg/s)  SphActuateTorqueX=off  SphActuateTorqueY=off  SphActuateTorqueZ=off  SphActuateTorque=off  SphTorqueActuationMode=NoTorque  SphMotionActuationMode=ComputedMotion  SphActuationFrame=BaseFrame  SphSensePosition=off  SphSenseVelocityX=off  SphSenseVelocityY=off  SphSenseVelocityZ=off  SphSenseVelocity=off  SphSenseAccelerationX=off  SphSenseAccelerationY=off  SphSenseAccelerationZ=off  SphSenseAcceleration=off  SphSenseTorqueX=off  SphSenseTorqueY=off  SphSenseTorqueZ=off  SphSenseTorqueForce=off  SphSensingFrame=BaseFrame  SphPositionTargetRotationMethod=None  SphPositionTargetRotationAngleUnits=deg  SphPositionTargetRotationStandardAxis=+Z  SphPositionTargetRotationAngle=0.0  SphPositionTargetRotationArbitraryAxis=[0 0 1]  SphPositionTargetFollAlignAxisA=+X  SphPositionTargetBaseAlignAxisA=+Y  SphPositionTargetFollAlignAxisB=+Y  SphPositionTargetBaseAlignAxisB=+Z  SphPositionTargetRotationMatrix=[1 0 0; 0 1 0; 0 0 1]  SphPositionTargetSpecify=off  SphPositionTargetPriority=High  SphVelocityTargetValue=[0 0 0]  SphVelocityTargetValueUnits=deg/s  SphVelocityTargetSpecify=off  SphVelocityTargetPriority=High  SphVelocityTargetInFollowerFrame=on  BlockFunction=simmechanics.library.joints.sixdof_joint
  Friction coeff : fl_lib/Physical Signals/Functions/PS Gain  gain=robot_floor_friction_coeff
  No friction : fl_lib/Physical Signals/Sources/PS Constant  constant=0
  PS Abs : fl_lib/Physical Signals/Nonlinear Operators/PS Abs
  PS-Simulink Converter : nesl_utility/PS-Simulink Converter  PhysicalDomain=network_engine_domain  SubClassName=ps_output  LeftPortType=input  RightPortType=output  PseudoPeriodic=off  Frequencies=[]  Unit=N  AffineConversion=off
  Saturation : Saturate  UpperLimit=+inf  LowerLimit=0
  Unary minus : fl_lib/Physical Signals/Functions/PS Gain  gain=-1
  X Lower Bound : fl_lib/Physical Signals/Nonlinear Operators/PS Max
  X Speed Gain : fl_lib/Physical Signals/Functions/PS Gain  gain=robot_floor_speed_gain
  X Switch : fl_lib/Physical Signals/Nonlinear Operators/PS Switch  Threshold=0
  X Upper Bound : fl_lib/Physical Signals/Nonlinear Operators/PS Min
  Y Lower Bound : fl_lib/Physical Signals/Nonlinear Operators/PS Max
  Y Speed Gain : fl_lib/Physical Signals/Functions/PS Gain  gain=robot_floor_speed_gain
  Y Switch : fl_lib/Physical Signals/Nonlinear Operators/PS Switch  Threshold=0
  Y Upper Bound : fl_lib/Physical Signals/Nonlinear Operators/PS Min
  Z Add : fl_lib/Physical Signals/Functions/PS Add
  Z Position Gain : fl_lib/Physical Signals/Functions/PS Gain  gain=robot_floor_position_gain
  Z Speed Gain : fl_lib/Physical Signals/Functions/PS Gain  gain=robot_floor_speed_gain
  Z Switch : fl_lib/Physical Signals/Nonlinear Operators/PS Switch  Threshold=0
  Contact : PMIOPort  Port=1  Side=Left
  Floor : PMIOPort  Port=2  Side=Right
  Z force : Outport
  wires:
  PS-Simulink Converter/1 -> Saturation/1
  Saturation/1 -> Z force/1
  connections:
  Floor/RConn1 -- 6-DOF Joint1/LConn1
  6-DOF Joint1/RConn1 -- Contact/RConn1
  No friction/RConn1 -- Y Switch/LConn1 -- Z Switch/LConn1 -- X Switch/LConn1
  Z Position Gain/RConn1 -- Z Add/LConn1
  Z Switch/LConn3 -- Z Add/RConn1 -- Friction coeff/LConn1 -- PS-Simulink Converter/LConn1
  Z Speed Gain/RConn1 -- Z Add/LConn2
  6-DOF Joint1/RConn5 -- Z Speed Gain/LConn1
  6-DOF Joint1/LConn4 -- Z Switch/RConn1
  Z Switch/LConn2 -- Z Position Gain/LConn1 -- 6-DOF Joint1/RConn4 -- X Switch/LConn2 -- Y Switch/LConn2
  Y Switch/RConn1 -- 6-DOF Joint1/LConn3
  Y Speed Gain/LConn1 -- 6-DOF Joint1/RConn3
  PS Abs/LConn1 -- Friction coeff/RConn1
  PS Abs/RConn1 -- Unary minus/LConn1 -- X Upper Bound/LConn2 -- Y Upper Bound/LConn2
  Y Upper Bound/RConn1 -- Y Lower Bound/LConn1
  Y Lower Bound/LConn2 -- Unary minus/RConn1 -- X Lower Bound/LConn2
  Y Lower Bound/RConn1 -- Y Switch/LConn3
  Y Upper Bound/LConn1 -- Y Speed Gain/RConn1
  X Speed Gain/LConn1 -- 6-DOF Joint1/RConn2
  X Upper Bound/LConn1 -- X Speed Gain/RConn1
  X Lower Bound/LConn1 -- X Upper Bound/RConn1
  X Switch/LConn3 -- X Lower Bound/RConn1
  X Switch/RConn1 -- 6-DOF Joint1/LConn2

== system robot_action/Right Leg/Floor model/Floor Model Front Left ==
  6-DOF Joint1 : sm_lib/Joints/6-DOF Joint  SenseConstraintForce=off  SenseConstraintForceX=off  SenseConstraintForceY=off  SenseConstraintForceZ=off  SenseConstraintTorque=off  SenseConstraintTorqueX=off  SenseConstraintTorqueY=off  SenseConstraintTorqueZ=off  SenseTotalForce=off  SenseTotalForceX=off  SenseTotalForceY=off  SenseTotalForceZ=off  SenseTotalTorque=off  SenseTotalTorqueX=off  SenseTotalTorqueY=off  SenseTotalTorqueZ=off  CompositeWrenchDir=FollowerOnBase  CompositeWrenchFrame=BaseFrame  PxEquilibriumPosition=0  PxEquilibriumPositionUnits=m  PxSpringStiffness=0  PxSpringStiffnessUnits=N/m  PxDampingCoefficient=0  PxDampingCoefficientUnits=N/(m/s)  PxTorqueActuationMode=InputTorque  PxMotionActuationMode=ComputedMotion  PxSensePosition=off  PxSenseVelocity=on  PxSenseAcceleration=off  PxSenseTorqueForce=off  PxPositionTargetValue=0  PxPositionTargetValueUnits=m  PxPositionTargetSpecify=off  PxPositionTargetPriority=High  PxVelocityTargetValue=0  PxVelocityTargetValueUnits=m/s  PxVelocityTargetSpecify=off  PxVelocityTargetPriority=High  PyEquilibriumPosition=0  PyEquilibriumPositionUnits=m  PySpringStiffness=0  PySpringStiffnessUnits=N/m  PyDampingCoefficient=0  PyDampingCoefficientUnits=N/(m/s)  PyTorqueActuationMode=InputTorque  PyMotionActuationMode=ComputedMotion  PySensePosition=off  PySenseVelocity=on  PySenseAcceleration=off  PySenseTorqueForce=off  PyPositionTargetValue=0  PyPositionTargetValueUnits=m  PyPositionTargetSpecify=off  PyPositionTargetPriority=High  PyVelocityTargetValue=0  PyVelocityTargetValueUnits=m/s  PyVelocityTargetSpecify=off  PyVelocityTargetPriority=High  PzEquilibriumPosition=0  PzEquilibriumPositionUnits=m  PzSpringStiffness=0  PzSpringStiffnessUnits=N/m  PzDampingCoefficient=0  PzDampingCoefficientUnits=N/(m/s)  PzTorqueActuationMode=InputTorque  PzMotionActuationMode=ComputedMotion  PzSensePosition=on  PzSenseVelocity=on  PzSenseAcceleration=off  PzSenseTorqueForce=off  PzPositionTargetValue=0  PzPositionTargetValueUnits=m  PzPositionTargetSpecify=off  PzPositionTargetPriority=High  PzVelocityTargetValue=0  PzVelocityTargetValueUnits=m/s  PzVelocityTargetSpecify=off  PzVelocityTargetPriority=High  SphDefPosRotationMethod=None  SphDefPosRotationAngleUnits=deg  SphDefPosRotationStandardAxis=+Z  SphDefPosRotationAngle=0.0  SphDefPosRotationArbitraryAxis=[0 0 1]  SphDefPosFollAlignAxisA=+X  SphDefPosBaseAlignAxisA=+Y  SphDefPosFollAlignAxisB=+Y  SphDefPosBaseAlignAxisB=+Z  SphDefPosRotationMatrix=[1 0 0; 0 1 0; 0 0 1]  SphEqPosRotationMethod=None  SphEqPosRotationAngleUnits=deg  SphEqPosRotationStandardAxis=+Z  SphEqPosRotationAngle=0.0  SphEqPosRotationArbitraryAxis=[0 0 1]  SphEqPosFollAlignAxisA=+X  SphEqPosBaseAlignAxisA=+Y  SphEqPosFollAlignAxisB=+Y  SphEqPosBaseAlignAxisB=+Z  SphEqPosRotationMatrix=[1 0 0; 0 1 0; 0 0 1]  SphSpringStiffness=0  SphSpringStiffnessUnits=N*m/deg  SphDampingCoefficient=0  SphDampingCoefficientUnits=N*m/(deg/s)  SphActuateTorqueX=off  SphActuateTorqueY=off  SphActuateTorqueZ=off  SphActuateTorque=off  SphTorqueActuationMode=NoTorque  SphMotionActuationMode=ComputedMotion  SphActuationFrame=BaseFrame  SphSensePosition=off  SphSenseVelocityX=off  SphSenseVelocityY=off  SphSenseVelocityZ=off  SphSenseVelocity=off  SphSenseAccelerationX=off  SphSenseAccelerationY=off  SphSenseAccelerationZ=off  SphSenseAcceleration=off  SphSenseTorqueX=off  SphSenseTorqueY=off  SphSenseTorqueZ=off  SphSenseTorqueForce=off  SphSensingFrame=BaseFrame  SphPositionTargetRotationMethod=None  SphPositionTargetRotationAngleUnits=deg  SphPositionTargetRotationStandardAxis=+Z  SphPositionTargetRotationAngle=0.0  SphPositionTargetRotationArbitraryAxis=[0 0 1]  SphPositionTargetFollAlignAxisA=+X  SphPositionTargetBaseAlignAxisA=+Y  SphPositionTargetFollAlignAxisB=+Y  SphPositionTargetBaseAlignAxisB=+Z  SphPositionTargetRotationMatrix=[1 0 0; 0 1 0; 0 0 1]  SphPositionTargetSpecify=off  SphPositionTargetPriority=High  SphVelocityTargetValue=[0 0 0]  SphVelocityTargetValueUnits=deg/s  SphVelocityTargetSpecify=off  SphVelocityTargetPriority=High  SphVelocityTargetInFollowerFrame=on  BlockFunction=simmechanics.library.joints.sixdof_joint
  Friction coeff : fl_lib/Physical Signals/Functions/PS Gain  gain=robot_floor_friction_coeff
  No friction : fl_lib/Physical Signals/Sources/PS Constant  constant=0
  PS Abs : fl_lib/Physical Signals/Nonlinear Operators/PS Abs
  PS-Simulink Converter : nesl_utility/PS-Simulink Converter  PhysicalDomain=network_engine_domain  SubClassName=ps_output  LeftPortType=input  RightPortType=output  PseudoPeriodic=off  Frequencies=[]  Unit=N  AffineConversion=off
  Saturation : Saturate  UpperLimit=+inf  LowerLimit=0
  Unary minus : fl_lib/Physical Signals/Functions/PS Gain  gain=-1
  X Lower Bound : fl_lib/Physical Signals/Nonlinear Operators/PS Max
  X Speed Gain : fl_lib/Physical Signals/Functions/PS Gain  gain=robot_floor_speed_gain
  X Switch : fl_lib/Physical Signals/Nonlinear Operators/PS Switch  Threshold=0
  X Upper Bound : fl_lib/Physical Signals/Nonlinear Operators/PS Min
  Y Lower Bound : fl_lib/Physical Signals/Nonlinear Operators/PS Max
  Y Speed Gain : fl_lib/Physical Signals/Functions/PS Gain  gain=robot_floor_speed_gain
  Y Switch : fl_lib/Physical Signals/Nonlinear Operators/PS Switch  Threshold=0
  Y Upper Bound : fl_lib/Physical Signals/Nonlinear Operators/PS Min
  Z Add : fl_lib/Physical Signals/Functions/PS Add
  Z Position Gain : fl_lib/Physical Signals/Functions/PS Gain  gain=robot_floor_position_gain
  Z Speed Gain : fl_lib/Physical Signals/Functions/PS Gain  gain=robot_floor_speed_gain
  Z Switch : fl_lib/Physical Signals/Nonlinear Operators/PS Switch  Threshold=0
  Contact : PMIOPort  Port=1  Side=Left
  Floor : PMIOPort  Port=2  Side=Right
  Z force : Outport
  wires:
  PS-Simulink Converter/1 -> Saturation/1
  Saturation/1 -> Z force/1
  connections:
  Floor/RConn1 -- 6-DOF Joint1/LConn1
  6-DOF Joint1/RConn1 -- Contact/RConn1
  No friction/RConn1 -- Y Switch/LConn1 -- Z Switch/LConn1 -- X Switch/LConn1
  Z Position Gain/RConn1 -- Z Add/LConn1
  Z Switch/LConn3 -- Z Add/RConn1 -- Friction coeff/LConn1 -- PS-Simulink Converter/LConn1
  Z Speed Gain/RConn1 -- Z Add/LConn2
  6-DOF Joint1/RConn5 -- Z Speed Gain/LConn1
  6-DOF Joint1/LConn4 -- Z Switch/RConn1
  Z Switch/LConn2 -- Z Position Gain/LConn1 -- 6-DOF Joint1/RConn4 -- X Switch/LConn2 -- Y Switch/LConn2
  Y Switch/RConn1 -- 6-DOF Joint1/LConn3
  Y Speed Gain/LConn1 -- 6-DOF Joint1/RConn3
  PS Abs/LConn1 -- Friction coeff/RConn1
  PS Abs/RConn1 -- Unary minus/LConn1 -- X Upper Bound/LConn2 -- Y Upper Bound/LConn2
  Y Upper Bound/RConn1 -- Y Lower Bound/LConn1
  Y Lower Bound/LConn2 -- Unary minus/RConn1 -- X Lower Bound/LConn2
  Y Lower Bound/RConn1 -- Y Switch/LConn3
  Y Upper Bound/LConn1 -- Y Speed Gain/RConn1
  X Speed Gain/LConn1 -- 6-DOF Joint1/RConn2
  X Upper Bound/LConn1 -- X Speed Gain/RConn1
  X Lower Bound/LConn1 -- X Upper Bound/RConn1
  X Switch/LConn3 -- X Lower Bound/RConn1
  X Switch/RConn1 -- 6-DOF Joint1/LConn2
